simulink model "external_memory_test"  (R2020b)
settings: Solver=FixedStepDiscrete  StartTime=0.0  StopTime=80  RelTol=1e-3
InitFcn:
  | Feature_Width = 64;
  | Feature_Height = 64;
  | Weight_Width = 3;
  | Weight_Height = 3;
  | external_memory_test_init;
values from neighbouring files (symbols this model uses):
  Burst_Length = Feature_Weight_Length    [external_memory_test_init.m]
  byPass = 1    [external_memory_test_init.m]
  Conv_Padding = 0    [external_memory_test_init.m]
  Conv_Stride = 1    [external_memory_test_init.m]
  DDR_Depth = Weight_Length + Feature_Length + outFeature_Length    [external_memory_test_init.m]
  ddrInitData = single((rand(1,DDR_Depth)))    [external_memory_test_init.m]
  Duty_Cycle = 0.5    [external_memory_test_init.m]
  Feature_Area = Feature_Width * Feature_Height    [external_memory_test_init.m]
  Feature_Length = Phase_In * Feature_Area    [external_memory_test_init.m]
  inChannel = 3    [external_memory_test_init.m]
  outChannel = 2    [external_memory_test_init.m]
  outFeature_Length = outFeature_Width * outFeature_Height * Phase_Out    [external_memory_test_init.m]
  Pool_Stride = 2    [external_memory_test_init.m]
  Pool_Width = 2    [external_memory_test_init.m]
  Tc = 1    [external_memory_test_init.m]
  Ti = 1    [external_memory_test_init.m]
  To = 1    [external_memory_test_init.m]
  Tr = 1    [external_memory_test_init.m]
  Weight_Length = Phase_In * Weight_Area * Phase_Out    [external_memory_test_init.m]
undefined symbols (not defined in the file or in its folder): Conv_Step, Pool_Step, sigbuilder_block
libraries: hdlsllib x85, simulink x44, visionhdlutilities x16
(part 2 of 6)

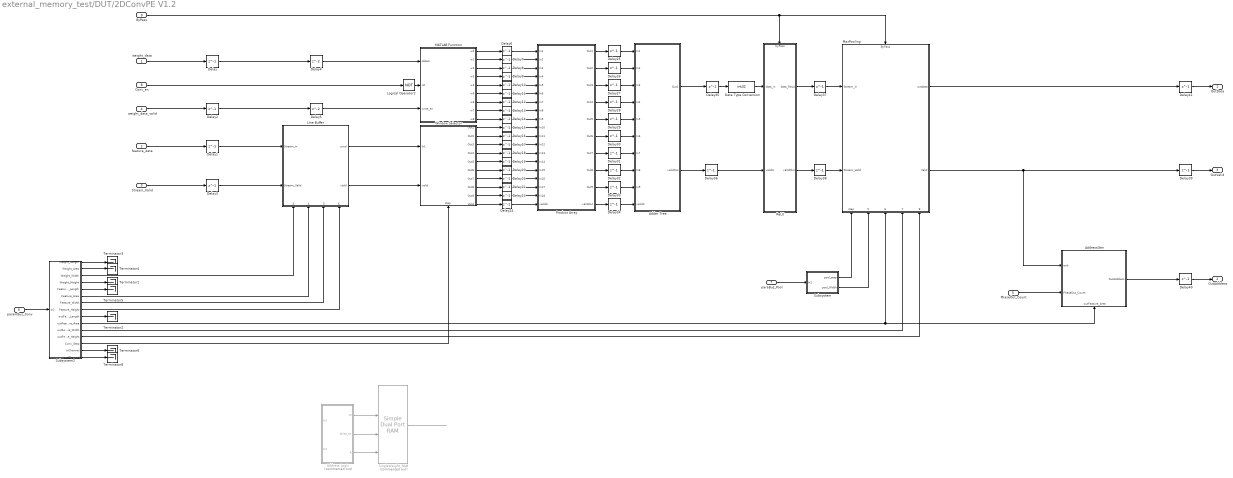
== system external_memory_test/DUT/2DConvPE V1.2 ==
  weight_data : Inport
  feature_data : Inport  Port=2
  Stream_Valid : Inport  Port=3
  weight_data_valid : Inport  Port=4
  PhaseOut_Count : Inport  Port=5
  paramBus_Conv : Inport  Port=6
  paraBus_Pool : Inport  Port=7
  Conv_en : Inport  Port=8
  ByPass : Inport  Port=9
  Adder Tree : Subsystem
  Address Logic : Subsystem  Commented=on
  AddressGen : Subsystem
      settings: PortSchema="{\"entries\":[{\"content\":{\"sides\":[{\"content\":{\"connectorIds\":[\"In1\",\"In2\"]},\"type\":\"ConnectorPlacement.EquallySpacedRectSide\",\"uuid\":\"84e29c71-0390-414b-ab77-a221de5de301\"},{\"content\":{\"connectorIds\":[\"Out1\"],\"side\":\"RIGHT\"},\"type\":\"ConnectorPlacement.EquallySpacedRectSide\",\"uuid\":\"58bcf278-1646-410a-a3e7-26ebbba1e273\"},{\"content\":{\"connectorIds\":[],\"side\":\"TOP\"},\"type\":\"ConnectorPlacement.EquallySpacedRectSide\",\"uuid\":\"d4babae5-c4b0-401f-9df6-cdd80e926352\"},{\"content\":{\"connectorIds\":[\"In3\"],\"side\":\"BOTTOM\"},\"type\":\"ConnectorPlacement.EquallySpacedRectSide\",\"uuid\":\"a08cab3a-dc4c-4404-aa4b-33dfd1f89102\"},{\"content\":{\"connectorIds\":[],\"side\":\"HIDDEN\"},\"type\":\"ConnectorPlacement.EquallySpacedRectSide\",\"uuid\":\"888452d7-95df-443f-995a-66331a7f8c73\"}]},\"type\":\"ConnectorPlacement.EquallySpacedConnector\",\"uuid\":\"691e5dfa-d85a-42aa-a608-f1539775aaa8\"}],\"packageUris\":[\"http://schema.mathworks.com/mf0/Connector/R2020b\"],\"version\":\"1.0\"}"
  Data Type Conversion : DataTypeConversion  OutDataTypeStr=int32
  Delay{,1..3,6..41} (40 alike) : Delay  DelayLength=1
  Delay4 : Delay
  Delay5 : Delay
  LIne Buffer : Subsystem
      settings: PortSchema="{\"entries\":[{\"content\":{\"sides\":[{\"content\":{\"connectorIds\":[\"In1\",\"In2\"]},\"type\":\"ConnectorPlacement.EquallySpacedRectSide\",\"uuid\":\"a250c848-7a40-462c-bfcf-0ff48046d99d\"},{\"content\":{\"connectorIds\":[\"Out1\",\"Out2\"],\"side\":\"RIGHT\"},\"type\":\"ConnectorPlacement.EquallySpacedRectSide\",\"uuid\":\"81aecf2d-6bfb-4d40-80c7-cfb89c921406\"},{\"content\":{\"connectorIds\":[],\"side\":\"TOP\"},\"type\":\"ConnectorPlacement.EquallySpacedRectSide\",\"uuid\":\"288ccc7a-b219-4526-a408-3d8b1082f4b0\"},{\"content\":{\"connectorIds\":[\"In3\",\"In4\",\"In5\",\"In6\"],\"side\":\"BOTTOM\"},\"type\":\"ConnectorPlacement.EquallySpacedRectSide\",\"uuid\":\"5d9529f5-ee70-4412-83ca-b280a2219284\"},{\"content\":{\"connectorIds\":[],\"side\":\"HIDDEN\"},\"type\":\"ConnectorPlacement.EquallySpacedRectSide\",\"uuid\":\"3d06d450-49b0-49ba-a273-690d97c3e8e1\"}]},\"type\":\"ConnectorPlacement.EquallySpacedConnector\",\"uuid\":\"b82e05d1-4695-4e04-9663-17698b30471b\"}],\"packageUris\":[\"http://schema.mathworks.com/mf0/Connector/R2020b\"],\"version\":\"1.0\"}"
  Logical Operator2 : Logic  Operator=NOT  AllPortsSameDT=off  OutDataTypeStr=boolean
  MATLAB Function : MATLAB Function  TreatAsAtomicUnit=on
  MaxPooling : Subsystem
      settings: PortSchema="{\"entries\":[{\"content\":{\"sides\":[{\"content\":{\"connectorIds\":[\"In1\",\"In2\"]},\"type\":\"ConnectorPlacement.EquallySpacedRectSide\",\"uuid\":\"8f082555-10a5-4426-9c6d-30ad9c9edc83\"},{\"content\":{\"connectorIds\":[\"Out1\",\"Out2\"],\"side\":\"RIGHT\"},\"type\":\"ConnectorPlacement.EquallySpacedRectSide\",\"uuid\":\"2f08e48d-98a7-49ef-9240-49e9a92f7835\"},{\"content\":{\"connectorIds\":[\"In3\"],\"side\":\"TOP\"},\"type\":\"ConnectorPlacement.EquallySpacedRectSide\",\"uuid\":\"9c785374-bdb9-47d6-a84c-95016a7dac24\"},{\"content\":{\"connectorIds\":[\"In4\",\"In5\",\"In6\",\"In7\",\"In8\"],\"side\":\"BOTTOM\"},\"type\":\"ConnectorPlacement.EquallySpacedRectSide\",\"uuid\":\"81220b33-16bc-4efc-91f7-9bf9738f949c\"},{\"content\":{\"connectorIds\":[],\"side\":\"HIDDEN\"},\"type\":\"ConnectorPlacement.EquallySpacedRectSide\",\"uuid\":\"99d22b10-fe8c-4c64-8a09-c433657226d7\"}]},\"type\":\"ConnectorPlacement.EquallySpacedConnector\",\"uuid\":\"f09d9050-86eb-4a30-82a2-eebdb84e68d3\"}],\"packageUris\":[\"http://schema.mathworks.com/mf0/Connector/R2020b\"],\"version\":\"1.0\"}"
  Product Array : Subsystem
  ReLU : Subsystem
      settings: PortSchema="{\"entries\":[{\"content\":{\"sides\":[{\"content\":{\"connectorIds\":[\"In1\",\"In2\"]},\"type\":\"ConnectorPlacement.EquallySpacedRectSide\",\"uuid\":\"abc19905-3b44-4985-b45b-942e5eaa1386\"},{\"content\":{\"connectorIds\":[\"Out1\",\"Out2\"],\"side\":\"RIGHT\"},\"type\":\"ConnectorPlacement.EquallySpacedRectSide\",\"uuid\":\"b0a86706-72e5-448b-9f1b-a0967f50aac9\"},{\"content\":{\"connectorIds\":[\"In3\"],\"side\":\"TOP\"},\"type\":\"ConnectorPlacement.EquallySpacedRectSide\",\"uuid\":\"df5d57b0-52e5-439f-8896-63a90ec5378c\"},{\"content\":{\"connectorIds\":[],\"side\":\"HIDDEN\"},\"type\":\"ConnectorPlacement.EquallySpacedRectSide\",\"uuid\":\"493b8843-365c-4ea1-b4d2-a52d72a7a785\"}]},\"type\":\"ConnectorPlacement.EquallySpacedConnector\",\"uuid\":\"755c5668-4a5f-4120-9a22-1155c417e52d\"}],\"packageUris\":[\"http://schema.mathworks.com/mf0/Connector/R2020b\"],\"version\":\"1.0\"}"
  SingleWeight_RAM : hdlsllib/HDL RAMs/Simple Dual Port RAM  Commented=on  ram_size=13
      settings: SourceProductName=HDL Coder
  Subsystem : Subsystem
  Subsystem2 : Subsystem
  Terminator{1..6,8} (7 alike) : Terminator
  Window Selector : Subsystem
      settings: PortSchema="{\"entries\":[{\"content\":{\"sides\":[{\"content\":{\"connectorIds\":[\"In1\",\"In2\"]},\"type\":\"ConnectorPlacement.EquallySpacedRectSide\",\"uuid\":\"2f98ee57-d732-418e-86bd-7acbaf2524e0\"},{\"content\":{\"connectorIds\":[\"Out1\",\"Out2\",\"Out3\",\"Out4\",\"Out5\",\"Out6\",\"Out7\",\"Out8\",\"Out9\",\"Out10\"],\"side\":\"RIGHT\"},\"type\":\"ConnectorPlacement.EquallySpacedRectSide\",\"uuid\":\"287ad403-178f-48f1-9791-2ccad363e9c6\"},{\"content\":{\"connectorIds\":[],\"side\":\"TOP\"},\"type\":\"ConnectorPlacement.EquallySpacedRectSide\",\"uuid\":\"a860ecae-5cde-45ef-a487-fdb4fb7390aa\"},{\"content\":{\"connectorIds\":[\"In3\"],\"side\":\"BOTTOM\"},\"type\":\"ConnectorPlacement.EquallySpacedRectSide\",\"uuid\":\"925435f5-0fb8-4a67-9f76-fe99b5b92634\"},{\"content\":{\"connectorIds\":[],\"side\":\"HIDDEN\"},\"type\":\"ConnectorPlacement.EquallySpacedRectSide\",\"uuid\":\"e6f3edac-a41a-4276-8ae6-cd8be9b02af9\"}]},\"type\":\"ConnectorPlacement.EquallySpacedConnector\",\"uuid\":\"0e32a9d0-da82-46c8-ab50-9de41c4380a9\"}],\"packageUris\":[\"http://schema.mathworks.com/mf0/Connector/R2020b\"],\"version\":\"1.0\"}"
  OutData : Outport
  OutAdddess : Outport  Port=2
  OutValid : Outport  Port=3
  wires:
  Delay/1 -> Delay4/1
  Address Logic/1(W) -> SingleWeight_RAM/2
  Address Logic/2(Write_en) -> SingleWeight_RAM/3
  Address Logic/3(R) -> SingleWeight_RAM/4
  SingleWeight_RAM/1 -> ?
  Conv_en/1 -> Logical Operator2/1
  Delay2/1 -> Delay5/1
  Logical Operator2/1 -> MATLAB Function/2(rst)
  AddressGen/1(OutAdddess) -> Delay40/1
  Adder Tree/1(Out1) -> Delay35/1
  Data Type Conversion/1 -> ReLU/1(data_in)
  ReLU/1(data_ReLU) -> Delay37/1
  PhaseOut_Count/1 -> AddressGen/2(PhaseOut_Count)
  ByPass/1 -> MaxPooling/3(ByPass), ReLU/3(byPass)
  MaxPooling/1(outdata) -> Delay41/1
  MaxPooling/2(Valid) -> Delay39/1, AddressGen/1(enb)
  paraBus_Pool/1 -> Subsystem/1(In1)
  Subsystem/1(pool_step) -> MaxPooling/4(step)
  Subsystem/2(pool_Width) -> MaxPooling/5(Window_Width)
  Subsystem2/11(outFeature_Width) -> MaxPooling/7(Feature_Width)
  Subsystem2/10(outFeature_Area) -> MaxPooling/6(Feature_Area), AddressGen/3(outFeature_Area)
  Subsystem2/12(outFeature_Height) -> MaxPooling/8(Feature_Height)
  paramBus_Conv/1 -> Subsystem2/1(In1)
  Subsystem2/14(inChannel) -> Terminator6/1
  Subsystem2/4(Weight_Height) -> Terminator1/1
  Subsystem2/9(outFeature_Length) -> Terminator2/1
  Subsystem2/13(Conv_Step) -> Window Selector/3(step)
  Subsystem2/1(Weight_Length) -> Terminator3/1
  Subsystem2/2(Weight_Area) -> Terminator4/1
  Subsystem2/5(Feature_Length) -> Terminator5/1
  Subsystem2/15(outChannel) -> Terminator8/1
  Adder Tree/2(validOut) -> Delay36/1
  ReLU/2(valildOut) -> Delay38/1
  Delay1/1 -> LIne Buffer/1(Stream_In)
  Delay3/1 -> LIne Buffer/2(Stream_Valid)
  Subsystem2/3(Weight_Width) -> LIne Buffer/3(Weight_Width)
  Subsystem2/6(Feature_Area) -> LIne Buffer/4(Feature_Area)
  Subsystem2/7(Feature_Width) -> LIne Buffer/5(Feature_Width)
  Subsystem2/8(Feature_Height) -> LIne Buffer/6(Feature_Height)
  LIne Buffer/1(pixel) -> Window Selector/1(In1)
  LIne Buffer/2(valid) -> Window Selector/2(valid)
  weight_data/1 -> Delay/1
  weight_data_valid/1 -> Delay2/1
  feature_data/1 -> Delay1/1
  Stream_Valid/1 -> Delay3/1
  Delay5/1 -> MATLAB Function/3(write_en)
  Delay4/1 -> MATLAB Function/1(dataIn)
  MATLAB Function/1(w0) -> Delay6/1
  Delay6/1 -> Product Array/1(In1)
  MATLAB Function/2(w1) -> Delay7/1
  Delay7/1 -> Product Array/2(In2)
  MATLAB Function/3(w2) -> Delay8/1
  Delay8/1 -> Product Array/3(In3)
  MATLAB Function/4(w3) -> Delay9/1
  Delay9/1 -> Product Array/4(In4)
  MATLAB Function/5(w4) -> Delay10/1
  Delay10/1 -> Product Array/5(In5)
  MATLAB Function/6(w5) -> Delay11/1
  Delay11/1 -> Product Array/6(In6)
  MATLAB Function/7(w6) -> Delay12/1
  Delay12/1 -> Product Array/7(In7)
  MATLAB Function/8(w7) -> Delay13/1
  Delay13/1 -> Product Array/8(In8)
  MATLAB Function/9(w8) -> Delay14/1
  Delay14/1 -> Product Array/9(In9)
  Window Selector/1(Out1) -> Delay15/1
  Delay15/1 -> Product Array/10(In10)
  Window Selector/2(Out2) -> Delay16/1
  Delay16/1 -> Product Array/11(In11)
  Window Selector/3(Out3) -> Delay17/1
  Delay17/1 -> Product Array/12(In12)
  Window Selector/4(Out4) -> Delay18/1
  Delay18/1 -> Product Array/13(In13)
  Window Selector/5(Out5) -> Delay19/1
  Delay19/1 -> Product Array/14(In14)
  Window Selector/6(Out6) -> Delay20/1
  Delay20/1 -> Product Array/15(In15)
  Window Selector/7(Out7) -> Delay21/1
  Delay21/1 -> Product Array/16(In16)
  Window Selector/8(Out8) -> Delay22/1
  Delay22/1 -> Product Array/17(In17)
  Window Selector/9(Out9) -> Delay23/1
  Delay23/1 -> Product Array/18(In18)
  Window Selector/10(Valid) -> Delay24/1
  Delay24/1 -> Product Array/19(validIn)
  Product Array/1(Out1) -> Delay25/1
  Delay25/1 -> Adder Tree/1(In1)
  Product Array/2(Out2) -> Delay26/1
  Product Array/3(Out3) -> Delay27/1
  Product Array/4(Out4) -> Delay28/1
  Product Array/5(Out5) -> Delay29/1
  Product Array/6(Out6) -> Delay30/1
  Product Array/7(Out7) -> Delay31/1
  Product Array/9(Out9) -> Delay33/1
  Product Array/8(Out8) -> Delay32/1
  Product Array/10(validOut) -> Delay34/1
  Delay26/1 -> Adder Tree/2(In2)
  Delay27/1 -> Adder Tree/3(In3)
  Delay28/1 -> Adder Tree/4(In4)
  Delay29/1 -> Adder Tree/5(In5)
  Delay30/1 -> Adder Tree/6(In6)
  Delay31/1 -> Adder Tree/7(In7)
  Delay32/1 -> Adder Tree/8(In8)
  Delay33/1 -> Adder Tree/9(In9)
  Delay34/1 -> Adder Tree/10(validIn)
  Delay35/1 -> Data Type Conversion/1
  Delay36/1 -> ReLU/2(validIn)
  Delay37/1 -> MaxPooling/1(Stream_In)
  Delay38/1 -> MaxPooling/2(Stream_Valid)
  Delay41/1 -> OutData/1
  Delay39/1 -> OutValid/1
  Delay40/1 -> OutAdddess/1

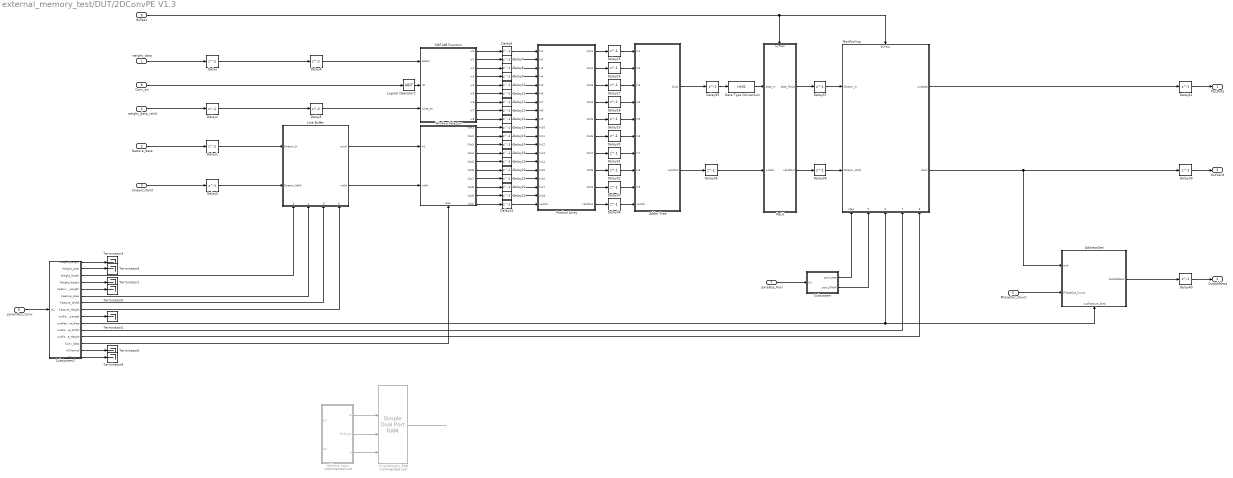
== system external_memory_test/DUT/2DConvPE V1.3 ==
  weight_data : Inport
  feature_data : Inport  Port=2
  Stream_Valid : Inport  Port=3
  weight_data_valid : Inport  Port=4
  PhaseOut_Count : Inport  Port=5
  paramBus_Conv : Inport  Port=6
  paraBus_Pool : Inport  Port=7
  Conv_en : Inport  Port=8
  ByPass : Inport  Port=9
  Adder Tree : Subsystem
  Address Logic : Subsystem  Commented=on
  AddressGen : Subsystem
      settings: PortSchema="{\"entries\":[{\"content\":{\"sides\":[{\"content\":{\"connectorIds\":[\"In1\",\"In2\"]},\"type\":\"ConnectorPlacement.EquallySpacedRectSide\",\"uuid\":\"84e29c71-0390-414b-ab77-a221de5de301\"},{\"content\":{\"connectorIds\":[\"Out1\"],\"side\":\"RIGHT\"},\"type\":\"ConnectorPlacement.EquallySpacedRectSide\",\"uuid\":\"58bcf278-1646-410a-a3e7-26ebbba1e273\"},{\"content\":{\"connectorIds\":[],\"side\":\"TOP\"},\"type\":\"ConnectorPlacement.EquallySpacedRectSide\",\"uuid\":\"d4babae5-c4b0-401f-9df6-cdd80e926352\"},{\"content\":{\"connectorIds\":[\"In3\"],\"side\":\"BOTTOM\"},\"type\":\"ConnectorPlacement.EquallySpacedRectSide\",\"uuid\":\"a08cab3a-dc4c-4404-aa4b-33dfd1f89102\"},{\"content\":{\"connectorIds\":[],\"side\":\"HIDDEN\"},\"type\":\"ConnectorPlacement.EquallySpacedRectSide\",\"uuid\":\"888452d7-95df-443f-995a-66331a7f8c73\"}]},\"type\":\"ConnectorPlacement.EquallySpacedConnector\",\"uuid\":\"691e5dfa-d85a-42aa-a608-f1539775aaa8\"}],\"packageUris\":[\"http://schema.mathworks.com/mf0/Connector/R2020b\"],\"version\":\"1.0\"}"
  Data Type Conversion : DataTypeConversion  OutDataTypeStr=int32
  Delay{,1..3,6..41} (40 alike) : Delay  DelayLength=1
  Delay4 : Delay
  Delay5 : Delay
  LIne Buffer : Subsystem
      settings: PortSchema="{\"entries\":[{\"content\":{\"sides\":[{\"content\":{\"connectorIds\":[\"In1\",\"In2\"]},\"type\":\"ConnectorPlacement.EquallySpacedRectSide\",\"uuid\":\"a250c848-7a40-462c-bfcf-0ff48046d99d\"},{\"content\":{\"connectorIds\":[\"Out1\",\"Out2\"],\"side\":\"RIGHT\"},\"type\":\"ConnectorPlacement.EquallySpacedRectSide\",\"uuid\":\"81aecf2d-6bfb-4d40-80c7-cfb89c921406\"},{\"content\":{\"connectorIds\":[],\"side\":\"TOP\"},\"type\":\"ConnectorPlacement.EquallySpacedRectSide\",\"uuid\":\"288ccc7a-b219-4526-a408-3d8b1082f4b0\"},{\"content\":{\"connectorIds\":[\"In3\",\"In4\",\"In5\",\"In6\"],\"side\":\"BOTTOM\"},\"type\":\"ConnectorPlacement.EquallySpacedRectSide\",\"uuid\":\"5d9529f5-ee70-4412-83ca-b280a2219284\"},{\"content\":{\"connectorIds\":[],\"side\":\"HIDDEN\"},\"type\":\"ConnectorPlacement.EquallySpacedRectSide\",\"uuid\":\"3d06d450-49b0-49ba-a273-690d97c3e8e1\"}]},\"type\":\"ConnectorPlacement.EquallySpacedConnector\",\"uuid\":\"b82e05d1-4695-4e04-9663-17698b30471b\"}],\"packageUris\":[\"http://schema.mathworks.com/mf0/Connector/R2020b\"],\"version\":\"1.0\"}"
  Logical Operator2 : Logic  Operator=NOT  AllPortsSameDT=off  OutDataTypeStr=boolean
  MATLAB Function : MATLAB Function  TreatAsAtomicUnit=on
  MaxPooling : Subsystem
      settings: PortSchema="{\"entries\":[{\"content\":{\"sides\":[{\"content\":{\"connectorIds\":[\"In1\",\"In2\"]},\"type\":\"ConnectorPlacement.EquallySpacedRectSide\",\"uuid\":\"8f082555-10a5-4426-9c6d-30ad9c9edc83\"},{\"content\":{\"connectorIds\":[\"Out1\",\"Out2\"],\"side\":\"RIGHT\"},\"type\":\"ConnectorPlacement.EquallySpacedRectSide\",\"uuid\":\"2f08e48d-98a7-49ef-9240-49e9a92f7835\"},{\"content\":{\"connectorIds\":[\"In3\"],\"side\":\"TOP\"},\"type\":\"ConnectorPlacement.EquallySpacedRectSide\",\"uuid\":\"9c785374-bdb9-47d6-a84c-95016a7dac24\"},{\"content\":{\"connectorIds\":[\"In4\",\"In5\",\"In6\",\"In7\",\"In8\"],\"side\":\"BOTTOM\"},\"type\":\"ConnectorPlacement.EquallySpacedRectSide\",\"uuid\":\"81220b33-16bc-4efc-91f7-9bf9738f949c\"},{\"content\":{\"connectorIds\":[],\"side\":\"HIDDEN\"},\"type\":\"ConnectorPlacement.EquallySpacedRectSide\",\"uuid\":\"99d22b10-fe8c-4c64-8a09-c433657226d7\"}]},\"type\":\"ConnectorPlacement.EquallySpacedConnector\",\"uuid\":\"f09d9050-86eb-4a30-82a2-eebdb84e68d3\"}],\"packageUris\":[\"http://schema.mathworks.com/mf0/Connector/R2020b\"],\"version\":\"1.0\"}"
  Product Array : Subsystem
  ReLU : Subsystem
      settings: PortSchema="{\"entries\":[{\"content\":{\"sides\":[{\"content\":{\"connectorIds\":[\"In1\",\"In2\"]},\"type\":\"ConnectorPlacement.EquallySpacedRectSide\",\"uuid\":\"abc19905-3b44-4985-b45b-942e5eaa1386\"},{\"content\":{\"connectorIds\":[\"Out1\",\"Out2\"],\"side\":\"RIGHT\"},\"type\":\"ConnectorPlacement.EquallySpacedRectSide\",\"uuid\":\"b0a86706-72e5-448b-9f1b-a0967f50aac9\"},{\"content\":{\"connectorIds\":[\"In3\"],\"side\":\"TOP\"},\"type\":\"ConnectorPlacement.EquallySpacedRectSide\",\"uuid\":\"df5d57b0-52e5-439f-8896-63a90ec5378c\"},{\"content\":{\"connectorIds\":[],\"side\":\"HIDDEN\"},\"type\":\"ConnectorPlacement.EquallySpacedRectSide\",\"uuid\":\"493b8843-365c-4ea1-b4d2-a52d72a7a785\"}]},\"type\":\"ConnectorPlacement.EquallySpacedConnector\",\"uuid\":\"755c5668-4a5f-4120-9a22-1155c417e52d\"}],\"packageUris\":[\"http://schema.mathworks.com/mf0/Connector/R2020b\"],\"version\":\"1.0\"}"
  SingleWeight_RAM : hdlsllib/HDL RAMs/Simple Dual Port RAM  Commented=on  ram_size=13
      settings: SourceProductName=HDL Coder
  Subsystem : Subsystem
  Subsystem2 : Subsystem
  Terminator{1..6,8} (7 alike) : Terminator
  Window Selector : Subsystem
      settings: PortSchema="{\"entries\":[{\"content\":{\"sides\":[{\"content\":{\"connectorIds\":[\"In1\",\"In2\"]},\"type\":\"ConnectorPlacement.EquallySpacedRectSide\",\"uuid\":\"2f98ee57-d732-418e-86bd-7acbaf2524e0\"},{\"content\":{\"connectorIds\":[\"Out1\",\"Out2\",\"Out3\",\"Out4\",\"Out5\",\"Out6\",\"Out7\",\"Out8\",\"Out9\",\"Out10\"],\"side\":\"RIGHT\"},\"type\":\"ConnectorPlacement.EquallySpacedRectSide\",\"uuid\":\"287ad403-178f-48f1-9791-2ccad363e9c6\"},{\"content\":{\"connectorIds\":[],\"side\":\"TOP\"},\"type\":\"ConnectorPlacement.EquallySpacedRectSide\",\"uuid\":\"a860ecae-5cde-45ef-a487-fdb4fb7390aa\"},{\"content\":{\"connectorIds\":[\"In3\"],\"side\":\"BOTTOM\"},\"type\":\"ConnectorPlacement.EquallySpacedRectSide\",\"uuid\":\"925435f5-0fb8-4a67-9f76-fe99b5b92634\"},{\"content\":{\"connectorIds\":[],\"side\":\"HIDDEN\"},\"type\":\"ConnectorPlacement.EquallySpacedRectSide\",\"uuid\":\"e6f3edac-a41a-4276-8ae6-cd8be9b02af9\"}]},\"type\":\"ConnectorPlacement.EquallySpacedConnector\",\"uuid\":\"0e32a9d0-da82-46c8-ab50-9de41c4380a9\"}],\"packageUris\":[\"http://schema.mathworks.com/mf0/Connector/R2020b\"],\"version\":\"1.0\"}"
  OutData : Outport
  OutAdddess : Outport  Port=2
  OutValid : Outport  Port=3
  wires:
  Delay/1 -> Delay4/1
  Address Logic/1(W) -> SingleWeight_RAM/2
  Address Logic/2(Write_en) -> SingleWeight_RAM/3
  Address Logic/3(R) -> SingleWeight_RAM/4
  SingleWeight_RAM/1 -> ?
  Conv_en/1 -> Logical Operator2/1
  Delay2/1 -> Delay5/1
  Logical Operator2/1 -> MATLAB Function/2(rst)
  AddressGen/1(OutAdddess) -> Delay40/1
  Adder Tree/1(Out1) -> Delay35/1
  Data Type Conversion/1 -> ReLU/1(data_in)
  ReLU/1(data_ReLU) -> Delay37/1
  PhaseOut_Count/1 -> AddressGen/2(PhaseOut_Count)
  ByPass/1 -> MaxPooling/3(ByPass), ReLU/3(byPass)
  MaxPooling/1(outdata) -> Delay41/1
  MaxPooling/2(Valid) -> Delay39/1, AddressGen/1(enb)
  paraBus_Pool/1 -> Subsystem/1(In1)
  Subsystem/1(pool_step) -> MaxPooling/4(step)
  Subsystem/2(pool_Width) -> MaxPooling/5(Window_Width)
  Subsystem2/11(outFeature_Width) -> MaxPooling/7(Feature_Width)
  Subsystem2/10(outFeature_Area) -> MaxPooling/6(Feature_Area), AddressGen/3(outFeature_Area)
  Subsystem2/12(outFeature_Height) -> MaxPooling/8(Feature_Height)
  paramBus_Conv/1 -> Subsystem2/1(In1)
  Subsystem2/14(inChannel) -> Terminator6/1
  Subsystem2/4(Weight_Height) -> Terminator1/1
  Subsystem2/9(outFeature_Length) -> Terminator2/1
  Subsystem2/13(Conv_Step) -> Window Selector/3(step)
  Subsystem2/1(Weight_Length) -> Terminator3/1
  Subsystem2/2(Weight_Area) -> Terminator4/1
  Subsystem2/5(Feature_Length) -> Terminator5/1
  Subsystem2/15(outChannel) -> Terminator8/1
  Adder Tree/2(validOut) -> Delay36/1
  ReLU/2(valildOut) -> Delay38/1
  Delay1/1 -> LIne Buffer/1(Stream_In)
  Delay3/1 -> LIne Buffer/2(Stream_Valid)
  Subsystem2/3(Weight_Width) -> LIne Buffer/3(Weight_Width)
  Subsystem2/6(Feature_Area) -> LIne Buffer/4(Feature_Area)
  Subsystem2/7(Feature_Width) -> LIne Buffer/5(Feature_Width)
  Subsystem2/8(Feature_Height) -> LIne Buffer/6(Feature_Height)
  LIne Buffer/1(pixel) -> Window Selector/1(In1)
  LIne Buffer/2(valid) -> Window Selector/2(valid)
  weight_data/1 -> Delay/1
  weight_data_valid/1 -> Delay2/1
  feature_data/1 -> Delay1/1
  Stream_Valid/1 -> Delay3/1
  Delay5/1 -> MATLAB Function/3(write_en)
  Delay4/1 -> MATLAB Function/1(dataIn)
  MATLAB Function/1(w0) -> Delay6/1
  Delay6/1 -> Product Array/1(In1)
  MATLAB Function/2(w1) -> Delay7/1
  Delay7/1 -> Product Array/2(In2)
  MATLAB Function/3(w2) -> Delay8/1
  Delay8/1 -> Product Array/3(In3)
  MATLAB Function/4(w3) -> Delay9/1
  Delay9/1 -> Product Array/4(In4)
  MATLAB Function/5(w4) -> Delay10/1
  Delay10/1 -> Product Array/5(In5)
  MATLAB Function/6(w5) -> Delay11/1
  Delay11/1 -> Product Array/6(In6)
  MATLAB Function/7(w6) -> Delay12/1
  Delay12/1 -> Product Array/7(In7)
  MATLAB Function/8(w7) -> Delay13/1
  Delay13/1 -> Product Array/8(In8)
  MATLAB Function/9(w8) -> Delay14/1
  Delay14/1 -> Product Array/9(In9)
  Window Selector/1(Out1) -> Delay15/1
  Delay15/1 -> Product Array/10(In10)
  Window Selector/2(Out2) -> Delay16/1
  Delay16/1 -> Product Array/11(In11)
  Window Selector/3(Out3) -> Delay17/1
  Delay17/1 -> Product Array/12(In12)
  Window Selector/4(Out4) -> Delay18/1
  Delay18/1 -> Product Array/13(In13)
  Window Selector/5(Out5) -> Delay19/1
  Delay19/1 -> Product Array/14(In14)
  Window Selector/6(Out6) -> Delay20/1
  Delay20/1 -> Product Array/15(In15)
  Window Selector/7(Out7) -> Delay21/1
  Delay21/1 -> Product Array/16(In16)
  Window Selector/8(Out8) -> Delay22/1
  Delay22/1 -> Product Array/17(In17)
  Window Selector/9(Out9) -> Delay23/1
  Delay23/1 -> Product Array/18(In18)
  Window Selector/10(Valid) -> Delay24/1
  Delay24/1 -> Product Array/19(validIn)
  Product Array/1(Out1) -> Delay25/1
  Delay25/1 -> Adder Tree/1(In1)
  Product Array/2(Out2) -> Delay26/1
  Product Array/3(Out3) -> Delay27/1
  Product Array/4(Out4) -> Delay28/1
  Product Array/5(Out5) -> Delay29/1
  Product Array/6(Out6) -> Delay30/1
  Product Array/7(Out7) -> Delay31/1
  Product Array/9(Out9) -> Delay33/1
  Product Array/8(Out8) -> Delay32/1
  Product Array/10(validOut) -> Delay34/1
  Delay26/1 -> Adder Tree/2(In2)
  Delay27/1 -> Adder Tree/3(In3)
  Delay28/1 -> Adder Tree/4(In4)
  Delay29/1 -> Adder Tree/5(In5)
  Delay30/1 -> Adder Tree/6(In6)
  Delay31/1 -> Adder Tree/7(In7)
  Delay32/1 -> Adder Tree/8(In8)
  Delay33/1 -> Adder Tree/9(In9)
  Delay34/1 -> Adder Tree/10(validIn)
  Delay35/1 -> Data Type Conversion/1
  Delay36/1 -> ReLU/2(validIn)
  Delay37/1 -> MaxPooling/1(Stream_In)
  Delay38/1 -> MaxPooling/2(Stream_Valid)
  Delay41/1 -> OutData/1
  Delay39/1 -> OutValid/1
  Delay40/1 -> OutAdddess/1

== system external_memory_test/DUT/Adder Tree ==
  In1 : Inport
  valid1 : Inport  Port=2
  In2 : Inport  Port=3
  valid2 : Inport  Port=4
  In3 : Inport  Port=5
  valid3 : Inport  Port=6
  In4 : Inport  Port=7
  valid4 : Inport  Port=8
  Add : Sum
  Add1 : Sum
  Add2 : Sum
  Logical Operator : Logic  Inputs=4  AllPortsSameDT=off  OutDataTypeStr=boolean
  Out1 : Outport
  outvalid : Outport  Port=2
  wires:
  Add/1 -> Add2/1
  In4/1 -> Add1/2
  Add2/1 -> Out1/1
  Add1/1 -> Add2/2
  In1/1 -> Add/1
  In3/1 -> Add1/1
  In2/1 -> Add/2
  valid1/1 -> Logical Operator/1
  valid2/1 -> Logical Operator/2
  valid3/1 -> Logical Operator/3
  valid4/1 -> Logical Operator/4
  Logical Operator/1 -> outvalid/1

== system external_memory_test/DUT/DDR_Access ==
  ram_read_data : Inport
  burst_len : Inport  Port=2
  burst_from_ddr : Inport  Port=3
  burst_start : Inport  Port=4
  axim_rd_data : Inport  Port=5
  axim_rd_s2m : Inport  Port=6
  axim_wr_s2m : Inport  Port=7
  Bus Creator : BusCreator  Inputs=3
  Bus Creator1 : BusCreator  Inputs=3
  Bus Selector1 : BusSelector  OutputSignals=wr_ready,wr_complete
  Bus Selector2 : BusSelector  OutputSignals=rd_aready,rd_dvalid
  DDR Read Conroller : MATLAB Function  TreatAsAtomicUnit=on
  DDR Write Conroller : MATLAB Function  TreatAsAtomicUnit=on
  EdgeDetection2 : Subsystem
  Logical Operator : Logic  IconShape=distinctive  AllPortsSameDT=off  OutDataTypeStr=boolean
  Logical Operator1 : Logic  IconShape=distinctive  AllPortsSameDT=off  OutDataTypeStr=boolean
  Logical Operator2 : Logic  Operator=NOT  IconShape=distinctive  AllPortsSameDT=off  OutDataTypeStr=boolean
  ram_wr_data : Outport  VectorParamsAs1DForOutWhenUnconnected=off
  ram_wr_addr : Outport  Port=2  VectorParamsAs1DForOutWhenUnconnected=off
  ram_wren : Outport  Port=3  VectorParamsAs1DForOutWhenUnconnected=off
  ram_rd_addr : Outport  Port=4  VectorParamsAs1DForOutWhenUnconnected=off
  ddr_read_done : Outport  Port=5  VectorParamsAs1DForOutWhenUnconnected=off
  ddr_write_done : Outport  Port=6  VectorParamsAs1DForOutWhenUnconnected=off
  axim_rd_m2s : Outport  Port=7  VectorParamsAs1DForOutWhenUnconnected=off
  axim_wr_data : Outport  Port=8  VectorParamsAs1DForOutWhenUnconnected=off
  axim_wr_m2s : Outport  Port=9  VectorParamsAs1DForOutWhenUnconnected=off
  wires:
  ram_read_data/1 -> axim_wr_data/1
  DDR Write Conroller/2(ddr_write_done) -> ddr_write_done/1
  DDR Read Conroller/3(ddr_read_done) -> ddr_read_done/1
  Logical Operator/1 -> DDR Read Conroller/2(start)
  Logical Operator2/1 -> Logical Operator1/2
  Logical Operator1/1 -> DDR Write Conroller/2(start)
  DDR Read Conroller/1(valid_out) -> ram_wren/1
  DDR Read Conroller/2(count_out) -> ram_wr_addr/1
  DDR Write Conroller/1(ram_addr) -> ram_rd_addr/1
  burst_from_ddr/1 -> Logical Operator/1, Logical Operator2/1
  axim_rd_data/1 -> ram_wr_data/1
  EdgeDetection2/1(Out1) -> Logical Operator/2, Logical Operator1/1
  burst_start/1 -> EdgeDetection2/1(In1)
  burst_len/1 -> DDR Write Conroller/1(burst_len), DDR Read Conroller/1(burst_len)
  axim_rd_s2m/1 -> Bus Selector2/1
  Bus Selector2/2 -> DDR Read Conroller/4(rd_dvalid)  "<rd_dvalid>"
  Bus Selector2/1 -> DDR Read Conroller/3(rd_aready)  "<rd_aready>"
  Bus Selector1/1 -> DDR Write Conroller/3(wr_ready)  "<wr_ready>"
  axim_wr_s2m/1 -> Bus Selector1/1
  DDR Read Conroller/5(rd_len) -> Bus Creator/2  "rd_len"
  DDR Read Conroller/4(rd_addr) -> Bus Creator/1  "rd_addr"
  Bus Creator/1 -> axim_rd_m2s/1
  DDR Read Conroller/6(rd_avalid) -> Bus Creator/3  "rd_avalid"
  DDR Write Conroller/5(wr_valid) -> Bus Creator1/3  "wr_valid"
  DDR Write Conroller/3(wr_addr) -> Bus Creator1/1  "wr_addr"
  DDR Write Conroller/4(wr_len) -> Bus Creator1/2  "wr_len"
  Bus Creator1/1 -> axim_wr_m2s/1
  Bus Selector1/2 -> DDR Write Conroller/4(wr_complete)  "<wr_complete>"

== system external_memory_test/DUT/Input Buffer ==
  ram_wr_data : Inport
  ram_wr_addr : Inport  Port=2
  ram_wr_en : Inport  Port=3
  ParamBus_Conv : Inport  Port=4
  BufferOut_en : Inport  Port=5
  Delay1 : Delay  DelayLength=1
  Delay2 : Delay  DelayLength=1
  Feature Buffer : Subsystem
  OutAddressLogic : Subsystem
      settings: PortSchema="{\"entries\":[{\"content\":{\"sides\":[{\"content\":{\"connectorIds\":[\"In1\",\"In2\",\"In3\",\"In4\",\"In5\",\"In6\",\"In7\"]},\"type\":\"ConnectorPlacement.EquallySpacedRectSide\",\"uuid\":\"80c0ec3c-65b3-4de5-aa3a-5b00fecd37ad\"},{\"content\":{\"connectorIds\":[\"Out1\",\"Out2\",\"Out3\",\"Out4\",\"Out5\"],\"side\":\"RIGHT\"},\"type\":\"ConnectorPlacement.EquallySpacedRectSide\",\"uuid\":\"b1c80772-a26a-47c2-b1eb-da8916c522e0\"},{\"content\":{\"connectorIds\":[\"In8\"],\"side\":\"TOP\"},\"type\":\"ConnectorPlacement.EquallySpacedRectSide\",\"uuid\":\"cc469776-1f0d-4664-a743-8cfa98e176ec\"},{\"content\":{\"connectorIds\":[],\"side\":\"HIDDEN\"},\"type\":\"ConnectorPlacement.EquallySpacedRectSide\",\"uuid\":\"373477cc-5f03-4dc7-9af7-ee6635f085f9\"}]},\"type\":\"ConnectorPlacement.EquallySpacedConnector\",\"uuid\":\"34946ddd-e540-4bf5-9b9a-fadd3b86bd62\"}],\"packageUris\":[\"http://schema.mathworks.com/mf0/Connector/R2020b\"],\"version\":\"1.0\"}"
  SeparateWrite : Subsystem
  Subsystem1 : Subsystem
  Weight Buffer : Subsystem
  weight_data : Outport
  feature_data : Outport  Port=2
  feature_data_valid : Outport  Port=3
  weight_data_valid : Outport  Port=4
  PhaseOut_Count : Outport  Port=5
  wires:
  Weight Buffer/1(ram_rd_data) -> weight_data/1
  Feature Buffer/1(ram_rd_data) -> feature_data/1
  ram_wr_addr/1 -> Weight Buffer/2(ram_wr_addr), SeparateWrite/2(In2)
  ram_wr_data/1 -> Weight Buffer/1(ram_wr_data), Feature Buffer/1(ram_wr_data)
  ram_wr_en/1 -> SeparateWrite/1(In1)
  SeparateWrite/1(Out1) -> Weight Buffer/3(ram_wr_en)
  SeparateWrite/2(Out2) -> Feature Buffer/2(ram_wr_addr)
  SeparateWrite/3(Out3) -> Feature Buffer/3(ram_wr_en)
  OutAddressLogic/2(featture_ram_rd_addr) -> Feature Buffer/4(ram_rd_addr)
  BufferOut_en/1 -> OutAddressLogic/8(Out_enable)
  OutAddressLogic/3(feature_data_valid) -> Delay1/1
  Delay1/1 -> feature_data_valid/1
  OutAddressLogic/1(weight_ram_rd_addr) -> Weight Buffer/4(ram_rd_addr)
  OutAddressLogic/4(weight_data_valid) -> Delay2/1
  Delay2/1 -> weight_data_valid/1
  OutAddressLogic/5(PhaseOut_Count) -> PhaseOut_Count/1
  Subsystem1/1(Weight_Length) -> SeparateWrite/3(Weight_Length), OutAddressLogic/1(Weight_Length)
  ParamBus_Conv/1 -> Subsystem1/1(In1)
  Subsystem1/2(Weight_Area) -> OutAddressLogic/2(Weight_Area)
  Subsystem1/3(Feature_Length) -> OutAddressLogic/3(Feature_Length)
  Subsystem1/4(Feature_Area) -> OutAddressLogic/4(Feature_Area)
  Subsystem1/5(Feature_Width) -> OutAddressLogic/5(Feature_Width)
  Subsystem1/6(Feature_Height) -> OutAddressLogic/6(Feature_Height)
  Subsystem1/7(outChannel) -> OutAddressLogic/7(outChannel)

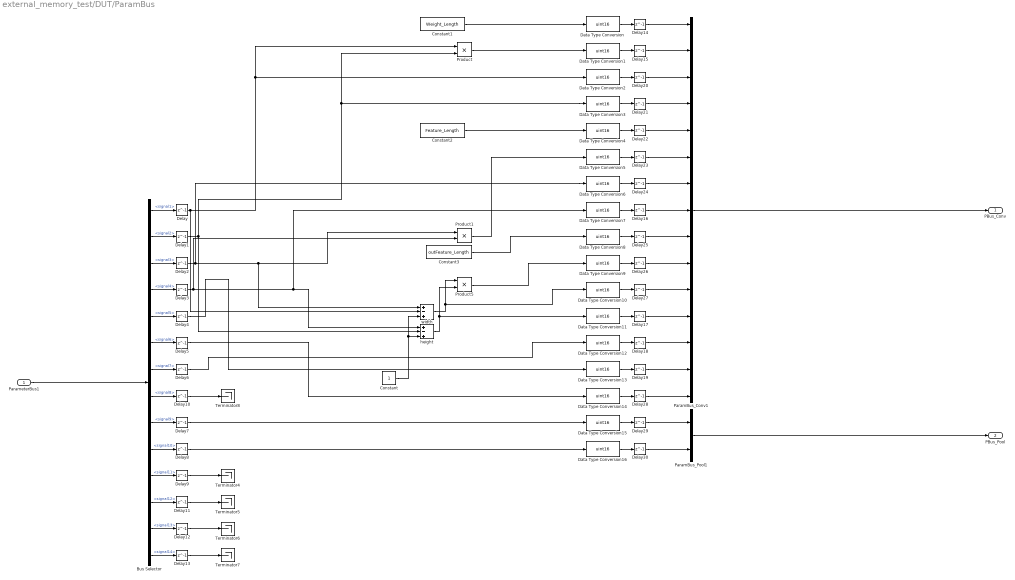
== system external_memory_test/DUT/ParamBus ==
  ParameterBus1 : Inport
  Bus Selector : BusSelector  OutputSignals=signal1,signal2,signal3,signal4,signal5,signal6,signal7,signal8,signal9,signal10,signal11,signal12,signal13,signal14
  Constant : Constant  OutDataTypeStr=uint32
  Constant1 : Constant  Value=Weight_Length  OutDataTypeStr=uint32
  Constant2 : Constant  Value=Feature_Length  OutDataTypeStr=uint32
  Constant3 : Constant  Value=outFeature_Length  OutDataTypeStr=uint32
  Data Type Conversion{,1..16} (17 alike) : DataTypeConversion  OutDataTypeStr=uint16
  Delay{,1..30} (31 alike) : Delay  DelayLength=1
  ParamBus_Conv1 : BusCreator  Inputs=15
  ParamBus_Pool1 : BusCreator  Inputs=2
  Product : Product
  Product1 : Product
  Product5 : Product
  Terminator{4..8} (5 alike) : Terminator
  height : Sum  Inputs=+-+
  width : Sum  Inputs=+-+
  PBus_Conv : Outport
  PBus_Pool : Outport  Port=2
  wires:
  ParameterBus1/1 -> Bus Selector/1
  Bus Selector/3 -> Delay2/1  "<signal3>"
  Bus Selector/4 -> Delay3/1  "<signal4>"
  Bus Selector/5 -> Delay4/1  "<signal5>"
  Bus Selector/6 -> Delay5/1  "<signal6>"
  Bus Selector/1 -> Delay/1  "<signal1>"
  Bus Selector/2 -> Delay1/1  "<signal2>"
  Bus Selector/7 -> Delay6/1  "<signal7>"
  Bus Selector/8 -> Delay10/1  "<signal8>"
  Bus Selector/9 -> Delay7/1  "<signal9>"
  Bus Selector/10 -> Delay8/1  "<signal10>"
  Bus Selector/11 -> Delay9/1  "<signal11>"
  Bus Selector/12 -> Delay11/1  "<signal12>"
  Bus Selector/13 -> Delay12/1  "<signal13>"
  Bus Selector/14 -> Delay13/1  "<signal14>"
  Delay/1 -> Data Type Conversion2/1, Product/1, width/2
  Delay1/1 -> Data Type Conversion3/1, Product/2, height/2
  Product/1 -> Data Type Conversion1/1
  Delay2/1 -> Product1/1, width/1, Data Type Conversion6/1
  Delay4/1 -> Data Type Conversion13/1
  Delay15/1 -> ParamBus_Conv1/2
  Delay14/1 -> ParamBus_Conv1/1
  Delay20/1 -> ParamBus_Conv1/3
  Delay21/1 -> ParamBus_Conv1/4
  Delay22/1 -> ParamBus_Conv1/5
  Delay23/1 -> ParamBus_Conv1/6
  Delay24/1 -> ParamBus_Conv1/7
  Delay16/1 -> ParamBus_Conv1/8
  Delay25/1 -> ParamBus_Conv1/9
  Delay26/1 -> ParamBus_Conv1/10
  Delay27/1 -> ParamBus_Conv1/11
  Delay17/1 -> ParamBus_Conv1/12
  Delay18/1 -> ParamBus_Conv1/13
  Delay19/1 -> ParamBus_Conv1/14
  Delay28/1 -> ParamBus_Conv1/15
  Product1/1 -> Data Type Conversion5/1
  Delay5/1 -> Data Type Conversion14/1
  Constant1/1 -> Data Type Conversion/1
  Delay7/1 -> Data Type Conversion15/1
  Delay8/1 -> Data Type Conversion16/1
  Delay29/1 -> ParamBus_Pool1/1
  Delay30/1 -> ParamBus_Pool1/2
  height/1 -> Product5/2, Data Type Conversion11/1
  Constant/1 -> height/3, width/3
  width/1 -> Data Type Conversion10/1, Product5/1
  Delay3/1 -> Data Type Conversion7/1, height/1, Product1/2
  Product5/1 -> Data Type Conversion9/1
  ParamBus_Conv1/1 -> PBus_Conv/1
  ParamBus_Pool1/1 -> PBus_Pool/1
  Delay6/1 -> Data Type Conversion12/1
  Delay9/1 -> Terminator4/1
  Delay11/1 -> Terminator5/1
  Delay12/1 -> Terminator6/1
  Delay13/1 -> Terminator7/1
  Delay10/1 -> Terminator8/1
  Constant2/1 -> Data Type Conversion4/1
  Constant3/1 -> Data Type Conversion8/1
  Data Type Conversion/1 -> Delay14/1
  Data Type Conversion14/1 -> Delay28/1
  Data Type Conversion12/1 -> Delay18/1
  Data Type Conversion13/1 -> Delay19/1
  Data Type Conversion1/1 -> Delay15/1
  Data Type Conversion2/1 -> Delay20/1
  Data Type Conversion3/1 -> Delay21/1
  Data Type Conversion4/1 -> Delay22/1
  Data Type Conversion5/1 -> Delay23/1
  Data Type Conversion6/1 -> Delay24/1
  Data Type Conversion10/1 -> Delay27/1
  Data Type Conversion7/1 -> Delay16/1
  Data Type Conversion8/1 -> Delay25/1
  Data Type Conversion9/1 -> Delay26/1
  Data Type Conversion11/1 -> Delay17/1
  Data Type Conversion15/1 -> Delay29/1
  Data Type Conversion16/1 -> Delay30/1

== system external_memory_test/DUT/outBuffer ==
  ram_wr_data : Inport
  ram_wr_addr : Inport  Port=2
  ram_wr_en : Inport  Port=3
  ram_rd_addr : Inport  Port=4
  Add : Sum
  Data Type Conversion : DataTypeConversion  OutDataTypeStr=int32
  Delay : Delay  DelayLength=1
  Delay1 : Delay  DelayLength=1
  Delay2 : Delay  DelayLength=1
  Out Buffer : Subsystem
  Switch : Switch
  ram_read_data : Outport
  wires:
  Out Buffer/1(ram_rd_data) -> Add/1, ram_read_data/1  "ram_read_data"
  ram_wr_addr/1 -> Delay/1, Switch/1
  ram_wr_data/1 -> Delay1/1
  ram_rd_addr/1 -> Switch/3
  ram_wr_en/1 -> Delay2/1, Switch/2
  Switch/1 -> Out Buffer/4(ram_rd_addr)
  Add/1 -> Data Type Conversion/1
  Delay/1 -> Out Buffer/2(ram_wr_addr)
  Data Type Conversion/1 -> Out Buffer/1(ram_wr_data)
  Delay1/1 -> Add/2
  Delay2/1 -> Out Buffer/3(ram_wr_en)

== system external_memory_test/InputSubsystem/Subsystem ==
  Constant18 : Constant  Value=Weight_Width  OutDataTypeStr=uint32  SampleTime=-1
  Constant19 : Constant  Value=outChannel  OutDataTypeStr=uint32  SampleTime=-1
  Constant20 : Constant  Value=Pool_Stride  OutDataTypeStr=uint32  SampleTime=-1
  Constant21 : Constant  Value=Conv_Stride  OutDataTypeStr=uint32  SampleTime=-1
  Constant22 : Constant  Value=Pool_Width  OutDataTypeStr=uint32  SampleTime=-1
  Constant23 : Constant  Value=Feature_Width  OutDataTypeStr=uint32  SampleTime=-1
  Constant24 : Constant  Value=Weight_Height  OutDataTypeStr=uint32  SampleTime=-1
  Constant25 : Constant  Value=inChannel  OutDataTypeStr=uint32  SampleTime=-1
  Constant26 : Constant  Value=Feature_Height  OutDataTypeStr=uint32  SampleTime=-1
  Constant27 : Constant  Value=Conv_Padding  OutDataTypeStr=uint32  SampleTime=-1
  Constant28 : Constant  Value=Ti  OutDataTypeStr=uint32  SampleTime=-1
  Constant29 : Constant  Value=To  OutDataTypeStr=uint32  SampleTime=-1
  Constant30 : Constant  Value=Tr  OutDataTypeStr=uint32  SampleTime=-1
  Constant31 : Constant  Value=Tc  OutDataTypeStr=uint32  SampleTime=-1
  weight_width : Outport
  Out2 : Outport  Port=2
  Out3 : Outport  Port=3
  Out4 : Outport  Port=4
  Out5 : Outport  Port=5
  Out6 : Outport  Port=6
  Out7 : Outport  Port=7
  Out8 : Outport  Port=8
  Out9 : Outport  Port=9
  Out10 : Outport  Port=10
  Out11 : Outport  Port=11
  Out12 : Outport  Port=12
  Out13 : Outport  Port=13
  Out14 : Outport  Port=14
  wires:
  Constant28/1 -> Out11/1
  Constant31/1 -> Out14/1
  Constant25/1 -> Out5/1
  Constant29/1 -> Out12/1
  Constant23/1 -> Out3/1
  Constant26/1 -> Out4/1
  Constant27/1 -> Out8/1
  Constant30/1 -> Out13/1
  Constant20/1 -> Out9/1
  Constant19/1 -> Out6/1
  Constant18/1 -> weight_width/1
  Constant24/1 -> Out2/1
  Constant21/1 -> Out7/1
  Constant22/1 -> Out10/1

== system external_memory_test/InputSubsystem/Subsystem1 ==
  Enable : EnablePort
  Signal Builder-Simulation : Subsystem  Tag=STV Subsys  LoadFcn=sigbuilder_block('load');  StartFcn=sigbuilder_block('start');  StopFcn=sigbuilder_block('stop');  ClipboardFcn=sigbuilder_block('clipboard');  mask(Sigbuilder block){tuvar=[0:10]}
      mask help: Simulink:masks:SigbuilderBlock_MD
      mask init:
      | if ~strcmp(get_param(bdroot(gcbh),'SimulationStatus'),'stopped') tuvar = sigbuilder_block('maskInit'); end
      settings: CopyFcn=sigbuilder_block('copy');  DeleteFcn=sigbuilder_block('delete');  ModelCloseFcn=sigbuilder_block('modelClose');  PreSaveFcn=sigbuilder_block('preSave');  PauseFcn=sigbuilder_block('pause');  ContinueFcn=sigbuilder_block('continue');  NameChangeFcn=sigbuilder_block('namechange');  OpenFcn=sigbuilder_block('open',[185.25 54.75 1047.75 640.5 ]);  CloseFcn=sigbuilder_block('close');
      mask Display: plot(0, 0, 100, 100,[2, 2, 32, 32, 2], [68, 8, 8, 68, 68],[32, 2], [38, 38], [32, 19, 2],[53, 60, 44], [32, 17, 17, 2],[16, 16, 31, 31]);txt = getActiveGroup(gcbh);text(2, 100, txt,'verticalAlignment', 'top');
  from_ddr_to_ram : Outport  VectorParamsAs1DForOutWhenUnconnected=off
  start : Outport  Port=2  VectorParamsAs1DForOutWhenUnconnected=off
  conv_en : Outport  Port=3
  wires:
  Signal Builder-Simulation/1(start) -> start/1
  Signal Builder-Simulation/2(from_ddr_to_ram) -> from_ddr_to_ram/1
  Signal Builder-Simulation/3(conv_en) -> conv_en/1

== system external_memory_test/OutputSubsystem/to_MATLAB ==
  ddr_init_done : Inport
  ramRdData : Inport  Port=2
  ramRdVal : Inport  Port=3
  load_done & rd_val : Logic  IconShape=distinctive  AllPortsSameDT=off  OutDataTypeStr=boolean
  to Matlab : Subsystem
  wires:
  ddr_init_done/1 -> load_done & rd_val/1
  load_done & rd_val/1 -> to Matlab/Enable
  ramRdVal/1 -> load_done & rd_val/2
  ramRdData/1 -> to Matlab/1(In1)

== system external_memory_test/DDR/wrLogic/Wr_control ==
  ddr_wr_rdy : Inport
  wr_enb : Inport  Port=2
  wr_len : Inport  Port=3
  AckGen : Subsystem
  MATLAB Function : MATLAB Function  TreatAsAtomicUnit=on
  Unit Delay : UnitDelay  SampleTime=-1  HasFrameUpgradeWarning=on
  valAddEnb : Outport  VectorParamsAs1DForOutWhenUnconnected=off
  axim_ack : Outport  Port=2  VectorParamsAs1DForOutWhenUnconnected=off
  ram_addr : Outport  Port=3  VectorParamsAs1DForOutWhenUnconnected=off
  wires:
  wr_enb/1 -> AckGen/2(wrEnb), MATLAB Function/1(axi_wr_en)
  AckGen/2(ValAddEnb) -> valAddEnb/1
  wr_len/1 -> MATLAB Function/2(axi_wr_length)
  AckGen/1(ack) -> Unit Delay/1
  MATLAB Function/1(wr_leng) -> AckGen/1(axiWrLen)
  Unit Delay/1 -> axim_ack/1, MATLAB Function/3(wr_ack)
  AckGen/3(ram_addr) -> ram_addr/1
  ddr_wr_rdy/1 -> AckGen/3(ddr_wr_rdy)

== system external_memory_test/DUT/2DConvPE V1.0/Adder Tree ==
  In1 : Inport
  In2 : Inport  Port=2
  In3 : Inport  Port=3
  In4 : Inport  Port=4
  In5 : Inport  Port=5
  In6 : Inport  Port=6
  In7 : Inport  Port=7
  In8 : Inport  Port=8
  In9 : Inport  Port=9
  validIn : Inport  Port=10
  Add{,1..6,10} (8 alike) : Sum
  Delay{1..9,35} (10 alike) : Delay  DelayLength=1
  Out1 : Outport
  validOut : Outport  Port=2
  wires:
  Add/1 -> Add4/1
  Add4/1 -> Add6/1
  Add10/1 -> Out1/1
  Add3/1 -> Add5/2
  Add2/1 -> Add5/1
  Add1/1 -> Add4/2
  Add6/1 -> Add10/1
  Add5/1 -> Add6/2
  Delay35/1 -> Add/1
  Delay1/1 -> Add/2
  Delay3/1 -> Add1/1
  Delay2/1 -> Add1/2
  Delay5/1 -> Add2/1
  Delay4/1 -> Add2/2
  Delay7/1 -> Add3/1
  Delay6/1 -> Add3/2
  In9/1 -> Delay8/1
  Delay8/1 -> Add10/2
  In8/1 -> Delay6/1
  In7/1 -> Delay7/1
  In6/1 -> Delay4/1
  In5/1 -> Delay5/1
  In4/1 -> Delay2/1
  In3/1 -> Delay3/1
  In2/1 -> Delay1/1
  In1/1 -> Delay35/1
  validIn/1 -> Delay9/1
  Delay9/1 -> validOut/1

== system external_memory_test/DUT/2DConvPE V1.0/Address Logic ==
  note: W/R_Address_Gen
  In1 : Inport
  In2 : Inport  Port=2
  " " : Subsystem
  Add : Sum  Inputs=+-
  Compare To Constant : simulink/Logic and Bit Operations/Compare To Constant  relop===  const=0  OutDataTypeStr=boolean
  Constant : Constant  OutDataTypeStr=uint32
  Delay : Delay  DelayLength=1
  Logical Operator1 : Logic  AllPortsSameDT=off  OutDataTypeStr=boolean
  Logical Operator2 : Logic  Operator=NOT  AllPortsSameDT=off  OutDataTypeStr=boolean
  Relational Operator : RelationalOperator  OutDataTypeStr=boolean  RndMeth=Simplest
  Weight_Counter : hdlsllib/Sources/HDL Counter  CountType=Free running  CountInit=0  CountStep=1  CountMax=2^15  CountFromType=Initial value  CountFrom=0  CountResetPort=on  CountLoadPort=off  CountEnbPort=on  CountDirPort=off  CountDataType=Unsigned  CountWordLen=32  CountFracLen=0  CountSampTime=1
  Weight_Interation_Counter : hdlsllib/Sources/HDL Counter  CountType=Free running  CountInit=0  CountStep=1  CountMax=2^15  CountFromType=Initial value  CountFrom=0  CountResetPort=on  CountLoadPort=off  CountEnbPort=on  CountDirPort=off  CountDataType=Unsigned  CountWordLen=32  CountFracLen=0  CountSampTime=1
  W : Outport
  Write_en : Outport  Port=2
  R : Outport  Port=3
  wires:
  Weight_Counter/1 -> " "/1(In1), Relational Operator/1
  Compare To Constant/1 -> Write_en/1, " "/2(In2)
  Delay/1 -> Logical Operator1/2, Logical Operator2/1, Weight_Counter/2
  Weight_Interation_Counter/1 -> Compare To Constant/1
  Constant/1 -> Add/2
  Logical Operator2/1 -> Weight_Interation_Counter/1
  " "/1(W) -> W/1
  Logical Operator1/1 -> Weight_Counter/1
  Relational Operator/1 -> Weight_Interation_Counter/2, Logical Operator1/1
  Add/1 -> Relational Operator/2
  In1/1 -> Delay/1
  In2/1 -> Add/1
  " "/2(R) -> R/1

== system external_memory_test/DUT/2DConvPE V1.0/AddressGen ==
  enb : Inport
  PhaseOut_Count : Inport  Port=2
  outFeature_Area : Inport  Port=3
  ADD : Sum
  Constant1 : Constant  Value=0  OutDataTypeStr=uint32  SampleTime=-1
  Constant2 : Constant  OutDataTypeStr=uint32  SampleTime=-1
  Minus : Sum  Inputs=+-
  OutAddress_Counter : hdlsllib/Sources/HDL Counter  CountType=Free running  CountInit=0  CountStep=1  CountMax=2^15  CountFromType=Initial value  CountFrom=0  CountResetPort=on  CountLoadPort=off  CountEnbPort=on  CountDirPort=off  CountDataType=Unsigned  CountWordLen=32  CountFracLen=0  CountSampTime=1
  Product : Product
  Relational Operator : RelationalOperator  OutDataTypeStr=boolean  RndMeth=Nearest
  Switch : Switch  Criteria=u2 ~= 0
  OutAdddess : Outport
  wires:
  Constant1/1 -> Switch/1
  Switch/1 -> Product/2
  OutAddress_Counter/1 -> Relational Operator/1, ADD/2
  outFeature_Area/1 -> Product/1, Minus/1
  Relational Operator/1 -> OutAddress_Counter/1
  Constant2/1 -> Minus/2
  Product/1 -> ADD/1
  ADD/1 -> OutAdddess/1
  Minus/1 -> Relational Operator/2
  enb/1 -> Switch/2, OutAddress_Counter/2
  PhaseOut_Count/1 -> Switch/3

== system external_memory_test/DUT/2DConvPE V1.0/LIne Buffer ==
  Stream_In : Inport
  Stream_Valid : Inport  Port=2
  Weight_Width : Inport  Port=3
  Feature_Area : Inport  Port=4
  Feature_Width : Inport  Port=5
  Feature_Height : Inport  Port=6
  Delay2 : Delay  DelayLength=1
  Line Buffer : Subsystem
  OutValidGen : Subsystem
  Terminator : Terminator
  pixel : Outport
  valid : Outport  Port=2
  wires:
  Feature_Area/1 -> Line Buffer/3(Feature_Area)
  Feature_Height/1 -> OutValidGen/3(Feature_Height)
  Line Buffer/3(shftEnable) -> Terminator/1
  Stream_In/1 -> Line Buffer/1(Stream_In)
  Line Buffer/1(pixel) -> Delay2/1
  Line Buffer/2(ctrl) -> OutValidGen/1(In1)
  Feature_Width/1 -> Line Buffer/4(Feature_Width)
  Stream_Valid/1 -> Line Buffer/2(Stream_Valid)
  Weight_Width/1 -> OutValidGen/2(Weight_Width)
  OutValidGen/1(valid) -> valid/1
  Delay2/1 -> pixel/1

== system external_memory_test/DUT/2DConvPE V1.0/MaxPooling ==
  Stream_In : Inport
  Stream_Valid : Inport  Port=2
  ByPass : Inport  Port=3
  step : Inport  Port=4
  Window_Width : Inport  Port=5
  Feature_Area : Inport  Port=6
  Feature_Width : Inport  Port=7
  Feature_Height : Inport  Port=8
  Comparator : Subsystem
  Constant : Constant  Value=0  OutDataTypeStr=int32
  Delay{,1..6,36} (8 alike) : Delay  DelayLength=1
  Line Buffer1 : Subsystem
  OutValidGen : Subsystem
  Switch : Switch  Criteria=u2 > Threshold
  Switch1 : Switch  Criteria=u2 > Threshold
  Terminator1 : Terminator
  dataSwitch : Switch  Criteria=u2 > Threshold
  validSwitch : Switch  Criteria=u2 > Threshold
  window Selector : Subsystem
  outdata : Outport
  Valid : Outport  Port=2
  wires:
  window Selector/3(Out3) -> Delay3/1
  OutValidGen/1(Out1) -> window Selector/2(valid)
  Feature_Width/1 -> Line Buffer1/4(Feature_Width)
  Line Buffer1/3(shftEnable) -> Terminator1/1
  Window_Width/1 -> OutValidGen/2(Window_Width)
  window Selector/5(Valid) -> Delay5/1
  window Selector/1(Out1) -> Delay/1
  Line Buffer1/1(pixel) -> Delay2/1
  Line Buffer1/2(ctrl) -> OutValidGen/1(ctrl)
  window Selector/2(Out2) -> Delay6/1
  window Selector/4(Out4) -> Delay4/1
  Feature_Area/1 -> Line Buffer1/3(Feature_Area)
  Feature_Height/1 -> OutValidGen/3(Feature_Height)
  step/1 -> window Selector/3(step)
  Delay1/1 -> validSwitch/1, Switch1/3
  Comparator/1(Out1) -> dataSwitch/3
  Delay36/1 -> dataSwitch/1, Switch/3
  ByPass/1 -> validSwitch/2, dataSwitch/2, Switch1/2, Switch/2
  dataSwitch/1 -> outdata/1
  validSwitch/1 -> Valid/1
  Constant/1 -> Switch1/1, Switch/1
  Switch/1 -> Line Buffer1/1(Stream_In)
  Switch1/1 -> Line Buffer1/2(Stream_Valid)
  Comparator/2(outvalid) -> validSwitch/3
  Stream_In/1 -> Delay36/1
  Stream_Valid/1 -> Delay1/1
  Delay2/1 -> window Selector/1(pixel)
  Delay/1 -> Comparator/1(In1)
  Delay5/1 -> Comparator/5(Valid)
  Delay4/1 -> Comparator/4(In4)
  Delay3/1 -> Comparator/3(In3)
  Delay6/1 -> Comparator/2(In2)

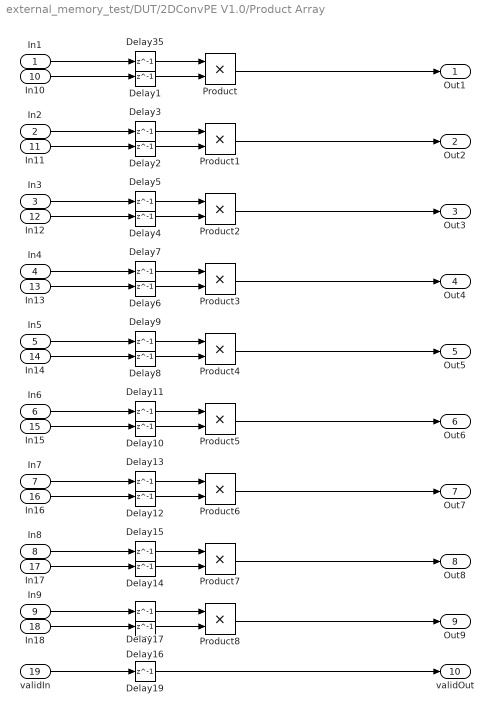
== system external_memory_test/DUT/2DConvPE V1.0/Product Array ==
  In1 : Inport
  In2 : Inport  Port=2
  In3 : Inport  Port=3
  In4 : Inport  Port=4
  In5 : Inport  Port=5
  In6 : Inport  Port=6
  In7 : Inport  Port=7
  In8 : Inport  Port=8
  In9 : Inport  Port=9
  In10 : Inport  Port=10
  In11 : Inport  Port=11
  In12 : Inport  Port=12
  In13 : Inport  Port=13
  In14 : Inport  Port=14
  In15 : Inport  Port=15
  In16 : Inport  Port=16
  In17 : Inport  Port=17
  In18 : Inport  Port=18
  validIn : Inport  Port=19
  Delay{1..17,19,35} (19 alike) : Delay  DelayLength=1
  Product{,1..8} (9 alike) : Product
  Out1 : Outport
  Out2 : Outport  Port=2
  Out3 : Outport  Port=3
  Out4 : Outport  Port=4
  Out5 : Outport  Port=5
  Out6 : Outport  Port=6
  Out7 : Outport  Port=7
  Out8 : Outport  Port=8
  Out9 : Outport  Port=9
  validOut : Outport  Port=10
  wires:
  Product/1 -> Out1/1
  In4/1 -> Delay7/1
  Product4/1 -> Out5/1
  In8/1 -> Delay15/1
  In17/1 -> Delay14/1
  In9/1 -> Delay17/1
  In12/1 -> Delay4/1
  In7/1 -> Delay13/1
  In1/1 -> Delay35/1
  In13/1 -> Delay6/1
  Product1/1 -> Out2/1
  In16/1 -> Delay12/1
  In10/1 -> Delay1/1
  In14/1 -> Delay8/1
  In18/1 -> Delay16/1
  Product8/1 -> Out9/1
  Product7/1 -> Out8/1
  In6/1 -> Delay11/1
  In2/1 -> Delay3/1
  In11/1 -> Delay2/1
  In15/1 -> Delay10/1
  In5/1 -> Delay9/1
  In3/1 -> Delay5/1
  Product3/1 -> Out4/1
  Product2/1 -> Out3/1
  Product5/1 -> Out6/1
  Product6/1 -> Out7/1
  validIn/1 -> Delay19/1
  Delay1/1 -> Product/2
  Delay35/1 -> Product/1
  Delay3/1 -> Product1/1
  Delay2/1 -> Product1/2
  Delay5/1 -> Product2/1
  Delay4/1 -> Product2/2
  Delay7/1 -> Product3/1
  Delay6/1 -> Product3/2
  Delay8/1 -> Product4/2
  Delay9/1 -> Product4/1
  Delay11/1 -> Product5/1
  Delay10/1 -> Product5/2
  Delay13/1 -> Product6/1
  Delay12/1 -> Product6/2
  Delay14/1 -> Product7/2
  Delay15/1 -> Product7/1
  Delay17/1 -> Product8/1
  Delay16/1 -> Product8/2
  Delay19/1 -> validOut/1

== system external_memory_test/DUT/2DConvPE V1.0/ReLU ==
  data_in : Inport
  validIn : Inport  Port=2
  byPass : Inport  Port=3
  Compare To Zero : simulink/Logic and Bit Operations/Compare To Zero  relop=>  OutDataTypeStr=boolean
  Constant : Constant  Value=0  OutDataTypeStr=int32
  Delay1 : Delay  DelayLength=1
  Delay36 : Delay  DelayLength=1
  Switch : Switch  Criteria=u2 > Threshold
  Switch1 : Switch  Criteria=u2 > Threshold
  data_ReLU : Outport
  valildOut : Outport  Port=2
  wires:
  Constant/1 -> Switch/3
  Delay36/1 -> Switch1/1, Switch/1, Compare To Zero/1
  Compare To Zero/1 -> Switch/2
  Switch/1 -> Switch1/3
  byPass/1 -> Switch1/2
  Switch1/1 -> data_ReLU/1
  Delay1/1 -> valildOut/1
  data_in/1 -> Delay36/1
  validIn/1 -> Delay1/1

== system external_memory_test/DUT/2DConvPE V1.0/Subsystem ==
  In1 : Inport
  Bus Selector : BusSelector  OutputSignals=signal1,signal2
  pool_step : Outport
  pool_Width : Outport  Port=2
  wires:
  Bus Selector/2 -> pool_Width/1  "<signal2>"
  Bus Selector/1 -> pool_step/1  "<signal1>"
  In1/1 -> Bus Selector/1
